simulink model "controller"  (R2018a)
settings: Solver=FixedStepAuto  StartTime=0.0  StopTime=inf  FixedStep=0.02  RelTol=1e-3  EnableMultiTasking=on
values from neighbouring files (symbols this model uses):
  data = zeros(2,4)    [LaneCal.m]
undefined symbols (not defined in the file or in its folder): control
libraries: simulink x21
settings Model: SimulationMode=accelerator  Creator=Owen  LastModifiedBy=shun.yang
settings SolverCC: AutoInsertRateTranBlk=on
settings DataIOCC: LimitDataPoints=on  SaveFormat=Array
settings OptimizationCC: EfficientMapNaN2IntZero=off  LifeSpan=inf  AccelVerboseBuild=on
settings DebuggingCC: SolverPrmCheckMsg=warning  SFUnexpectedBacktrackingDiag=warning  SFNoUnconditionalDefaultTransitionDiag=warning  SFExecutionAtInitializationDiag=none
settings HardwareCC: ProdBitPerPointer=32  ProdBitPerSizeT=32  ProdBitPerPtrDiffT=32  ProdLargestAtomicFloat=None  ProdIntDivRoundTo=Undefined  ProdEndianess=Unspecified  ProdWordSize=32  ProdHWDeviceType=32-bit Generic  TargetBitPerPointer=64  TargetBitPerSizeT=64  TargetBitPerPtrDiffT=64  TargetLongLongMode=on  TargetIntDivRoundTo=Zero  TargetEndianess=LittleEndian  TargetWordSize=64  TargetHWDeviceType=MATLAB Host  ProdEqTarget=off
settings ModelReferenceCC: PropagateSignalLabelsOutOfModel=off
settings SFSimCC: SimCustomInitializer=initTORCSLink();  SimCustomTerminator=terminateTORCSLink();  SimUserSources=TORCSLink.c  SimBuildMode=sf_nonincremental_build  SimGenImportedTypeDefs=on
settings CodeAppCC: MaxIdLength=128  StateflowObjectComments=on
settings GRTTargetCC: TargetLangStandard=C89/C90 (ANSI)  GeneratePreprocessorConditionals=Disable all  CombineOutputUpdateFcns=off  GRTInterface=on
settings ConfigComp: CovMetricSettings=dw  CovHtmlReporting=on  CovSaveCumulativeToWorkspaceVar=on  CovSaveSingleToWorkspaceVar=on  CovExternalEMLEnable=off  CovSFcnEnable=off

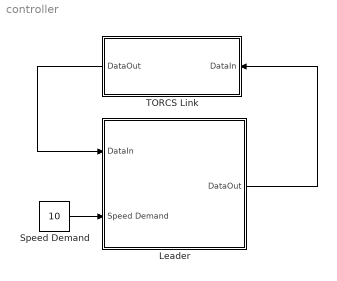
== system controller ==
  Leader : Subsystem
  Speed Demand : Constant  Value=10
  TORCS Link : Subsystem  LoadFcn=|  InitFcn=|
      LoadFcn=|
      | load VehicleBusses.mat;
      | src = 'TORCSLink.c';
      | init = 'initTORCSLink();';
      | term = 'terminateTORCSLink();';
      | simSrc = get_param(gcs,'SimUserSources');
      | simInit = get_param(gcs,'SimCustomInitializer');
      | simTerm = get_param(gcs,'SimCustomTerminator');
      | 
      | if isempty(strfind(simSrc,src))
      |   fprintf('Adding %s to Custom Sources\n', src);
      |   set_param(gcs,'SimUserSources', [simSrc 10 src]);
      | end
      | 
      | if isempty(strfind(simInit,init))
      |   fprintf('Adding %s to Custom Initialisation Code\n', init);
      |   set_param(gcs,'SimCustomInitializer', [simInit 10 init]);
      | end
      | 
      | if isempty(strfind(simTerm,term))
      |   fprintf('Adding %s to Custom Termination Code\n', term);
      |   set_param(gcs,'SimCustomTerminator', [simTerm 10 term]);
      | end
      | 
      | if isunix
      |     libs = 'librt.so';
      |     simLibs = get_param(gcs,'SimUserLibraries');
      | 
      |     if isempty(strfind(simLibs,libs))
      |       fprintf('Adding %s to Custom Libraries\n', libs);
      |       set_param(gcs,'SimUserLibraries', [simLibs 10 libs]);
      |     end
      | else
      |    set_param(gcs,'SimUserLibraries', '');
      | end
      | 
      | clear src init term simSrc simInit simTerm libs simLibs;
      InitFcn=|
      | load VehicleBusses.mat;
      | src = 'TORCSLink.c';
      | init = 'initTORCSLink();';
      | term = 'terminateTORCSLink();';
      | simSrc = get_param(gcs,'SimUserSources');
      | simInit = get_param(gcs,'SimCustomInitializer');
      | simTerm = get_param(gcs,'SimCustomTerminator');
      | 
      | if isempty(strfind(simSrc,src))
      |   fprintf('Adding %s to Custom Sources\n', src);
      |   set_param(gcs,'SimUserSources', [simSrc 10 src]);
      | end
      | 
      | if isempty(strfind(simInit,init))
      |   fprintf('Adding %s to Custom Initialisation Code\n', init);
      |   set_param(gcs,'SimCustomInitializer', [simInit 10 init]);
      | end
      | 
      | if isempty(strfind(simTerm,term))
      |   fprintf('Adding %s to Custom Termination Code\n', term);
      |   set_param(gcs,'SimCustomTerminator', [simTerm 10 term]);
      | end
      | 
      | if isunix
      |     libs = 'librt.so';
      |     simLibs = get_param(gcs,'SimUserLibraries');
      | 
      |     if isempty(strfind(simLibs,libs))
      |       fprintf('Adding %s to Custom Libraries\n', libs);
      |       set_param(gcs,'SimUserLibraries', [simLibs 10 libs]);
      |     end
      | else
      |    set_param(gcs,'SimUserLibraries', '');
      | end
      | 
      | clear src init term simSrc simInit simTerm libs simLibs;
  wires:
  TORCS Link/1(DataOut) -> Leader/1(DataIn)
  Speed Demand/1 -> Leader/2(Speed Demand)
  Leader/1(DataOut) -> TORCS Link/1(DataIn)

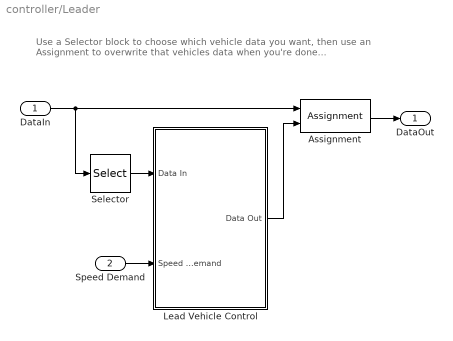
== system controller/Leader ==
  note: Use a Selector block to choose which vehicle data you want,
      | then use an Assignment to overwrite that vehicles data when you're done...
  DataIn : Inport
  Speed Demand : Inport  Port=2
  Assignment : Assignment  DiagnosticForDimensions=Warning  IndexOptions=Index vector (dialog)  Indices=1  OutputSizes=1
  Lead Vehicle Control : Subsystem  InitFcn=run Inita.m
  Selector : Selector  InputPortWidth=10  IndexOptions=Index vector (dialog)  Indices=1  OutputSizes=1
  DataOut : Outport
  wires:
  Speed Demand/1 -> Lead Vehicle Control/2(Speed Demand)
  DataIn/1 -> Selector/1, Assignment/1
  Selector/1 -> Lead Vehicle Control/1(Data In)
  Assignment/1 -> DataOut/1
  Lead Vehicle Control/1(Data Out) -> Assignment/2

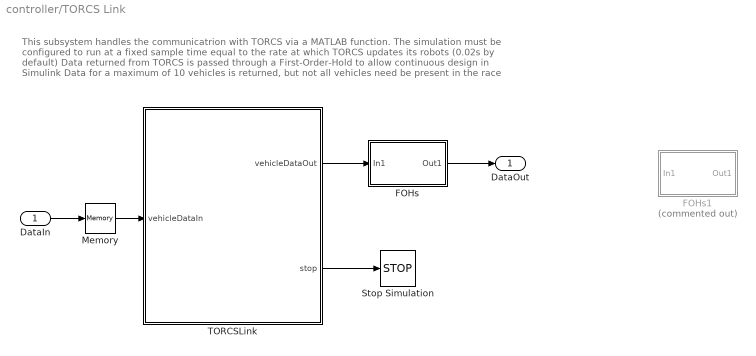
== system controller/TORCS Link ==
  note: This subsystem handles the communicatrion with TORCS via a MATLAB function.
      | The simulation must be configured to run at a fixed sample time equal to the rate at which TORCS updates its robots (0.02s by default)
      | Data returned from TORCS is passed through a First-Order-Hold to allow continuous design in Simulink
      | Data for a maximum of 10 vehicles is returned, but not all vehicles need be present in the race
  DataIn : Inport
  FOHs : Subsystem  TreatAsAtomicUnit=on
  FOHs1 : Subsystem  Commented=on  TreatAsAtomicUnit=on
  Memory : Memory
  Stop Simulation : Stop
  TORCSLink : MATLAB Function  TreatAsAtomicUnit=on
  DataOut : Outport
  wires:
  Memory/1 -> TORCSLink/1(vehicleDataIn)
  DataIn/1 -> Memory/1
  TORCSLink/2(stop) -> Stop Simulation/1
  TORCSLink/1(vehicleDataOut) -> FOHs/1(In1)
  FOHs/1(Out1) -> DataOut/1

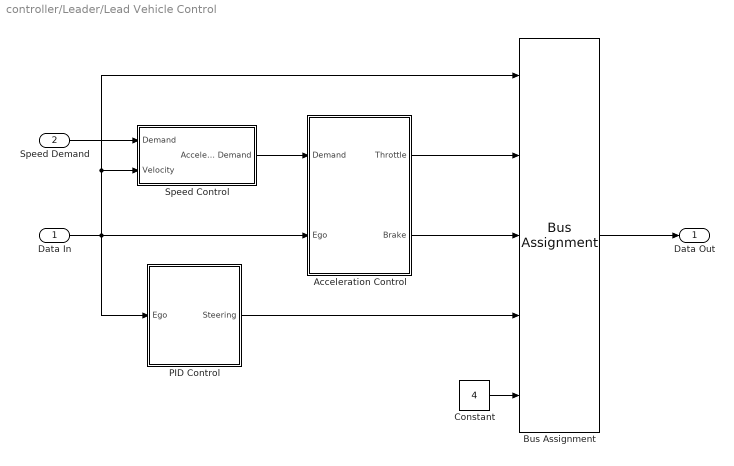
== system controller/Leader/Lead Vehicle Control ==
  Data In : Inport
  Speed Demand : Inport  Port=2
  Acceleration Control : Subsystem
  Bus Assignment : BusAssignment  AssignedSignals=control.throttle,control.brake,control.steering,control.gear
  Constant : Constant  Value=4  OutDataTypeStr=int32
  PID Control : Subsystem
  Speed Control : Subsystem
  Data Out : Outport
  wires:
  Speed Demand/1 -> Speed Control/1(Demand)
  Bus Assignment/1 -> Data Out/1
  Speed Control/1(Acceleration Demand) -> Acceleration Control/1(Demand)
  Data In/1 -> Acceleration Control/2(Ego), PID Control/1(Ego), Speed Control/2(Velocity), Bus Assignment/1
  Acceleration Control/2(Brake) -> Bus Assignment/3
  Acceleration Control/1(Throttle) -> Bus Assignment/2
  Constant/1 -> Bus Assignment/5
  PID Control/1(Steering) -> Bus Assignment/4

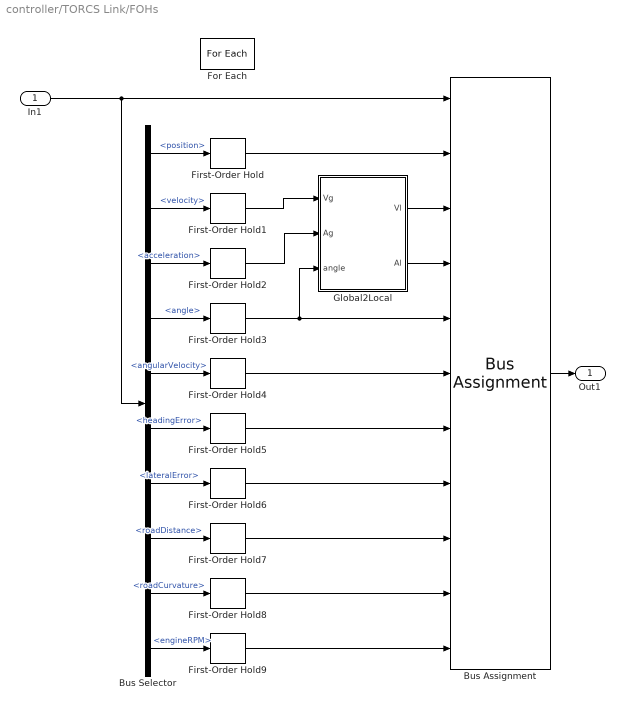
== system controller/TORCS Link/FOHs ==
  In1 : Inport  Partition=on  PartitionDimension=1  PartitionWidth=1  PartitionOffset=0
  Bus Assignment : BusAssignment  AssignedSignals=data.position,data.velocity,data.acceleration,data.angle,data.angularVelocity,data.headingError,data.lateralError,data.roadDistance,data.roadCurvature,data.engineRPM
  Bus Selector : BusSelector  OutputSignals=data.position,data.velocity,data.acceleration,data.angle,data.angularVelocity,data.headingError,data.lateralError,data.roadDistance,data.roadCurvature,data.engineRPM
  First-Order Hold{,1..9} (10 alike) : simulink/Discrete/First-Order Hold  DisableCoverage=on  Ts=0.02
      settings: SourceProductName=Simulink  SourceProductBaseCode=SL
  For Each : ForEach  DisableCoverage=on  IndexMode=One-based
  Global2Local : MATLAB Function  TreatAsAtomicUnit=on
  Out1 : Outport  ConcatenationDimension=1
  wires:
  Bus Assignment/1 -> Out1/1
  Bus Selector/10 -> First-Order Hold9/1  "<engineRPM>"
  Bus Selector/9 -> First-Order Hold8/1  "<roadCurvature>"
  Bus Selector/8 -> First-Order Hold7/1  "<roadDistance>"
  Bus Selector/7 -> First-Order Hold6/1  "<lateralError>"
  Bus Selector/6 -> First-Order Hold5/1  "<headingError>"
  Bus Selector/5 -> First-Order Hold4/1  "<angularVelocity>"
  Bus Selector/3 -> First-Order Hold2/1  "<acceleration>"
  Bus Selector/2 -> First-Order Hold1/1  "<velocity>"
  Bus Selector/1 -> First-Order Hold/1  "<position>"
  In1/1 -> Bus Assignment/1, Bus Selector/1
  Bus Selector/4 -> First-Order Hold3/1  "<angle>"
  First-Order Hold3/1 -> Global2Local/3(angle), Bus Assignment/5
  First-Order Hold4/1 -> Bus Assignment/6
  First-Order Hold5/1 -> Bus Assignment/7
  First-Order Hold6/1 -> Bus Assignment/8
  First-Order Hold7/1 -> Bus Assignment/9
  First-Order Hold8/1 -> Bus Assignment/10
  First-Order Hold9/1 -> Bus Assignment/11
  First-Order Hold1/1 -> Global2Local/1(Vg)
  First-Order Hold2/1 -> Global2Local/2(Ag)
  First-Order Hold/1 -> Bus Assignment/2
  Global2Local/2(Al) -> Bus Assignment/4
  Global2Local/1(Vl) -> Bus Assignment/3

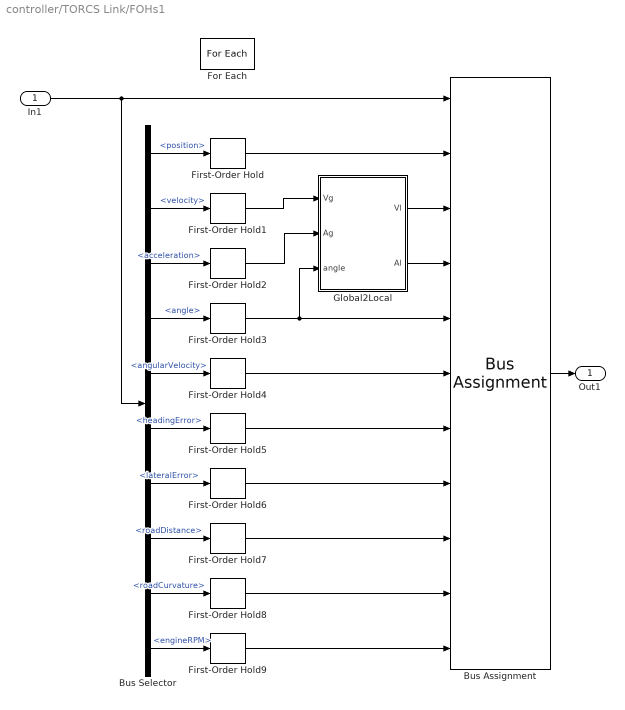
== system controller/TORCS Link/FOHs1 ==
  In1 : Inport  Partition=on  PartitionDimension=1  PartitionWidth=1  PartitionOffset=0
  Bus Assignment : BusAssignment  AssignedSignals=data.position,data.velocity,data.acceleration,data.angle,data.angularVelocity,data.headingError,data.lateralError,data.roadDistance,data.roadCurvature,data.engineRPM
  Bus Selector : BusSelector  OutputSignals=data.position,data.velocity,data.acceleration,data.angle,data.angularVelocity,data.headingError,data.lateralError,data.roadDistance,data.roadCurvature,data.engineRPM
  First-Order Hold{,1..9} (10 alike) : simulink/Discrete/First-Order Hold  DisableCoverage=on  Ts=0.1
      settings: SourceProductName=Simulink  SourceProductBaseCode=SL
  For Each : ForEach  DisableCoverage=on  IndexMode=One-based
  Global2Local : MATLAB Function  TreatAsAtomicUnit=on
  Out1 : Outport  ConcatenationDimension=1
  wires:
  Global2Local/1(Vl) -> Bus Assignment/3
  Global2Local/2(Al) -> Bus Assignment/4
  First-Order Hold/1 -> Bus Assignment/2
  First-Order Hold2/1 -> Global2Local/2(Ag)
  First-Order Hold1/1 -> Global2Local/1(Vg)
  First-Order Hold9/1 -> Bus Assignment/11
  First-Order Hold8/1 -> Bus Assignment/10
  First-Order Hold7/1 -> Bus Assignment/9
  First-Order Hold6/1 -> Bus Assignment/8
  First-Order Hold5/1 -> Bus Assignment/7
  First-Order Hold4/1 -> Bus Assignment/6
  First-Order Hold3/1 -> Bus Assignment/5, Global2Local/3(angle)
  Bus Selector/4 -> First-Order Hold3/1  "<angle>"
  In1/1 -> Bus Selector/1, Bus Assignment/1
  Bus Selector/1 -> First-Order Hold/1  "<position>"
  Bus Selector/2 -> First-Order Hold1/1  "<velocity>"
  Bus Selector/3 -> First-Order Hold2/1  "<acceleration>"
  Bus Selector/5 -> First-Order Hold4/1  "<angularVelocity>"
  Bus Selector/6 -> First-Order Hold5/1  "<headingError>"
  Bus Selector/7 -> First-Order Hold6/1  "<lateralError>"
  Bus Selector/8 -> First-Order Hold7/1  "<roadDistance>"
  Bus Selector/9 -> First-Order Hold8/1  "<roadCurvature>"
  Bus Selector/10 -> First-Order Hold9/1  "<engineRPM>"
  Bus Assignment/1 -> Out1/1

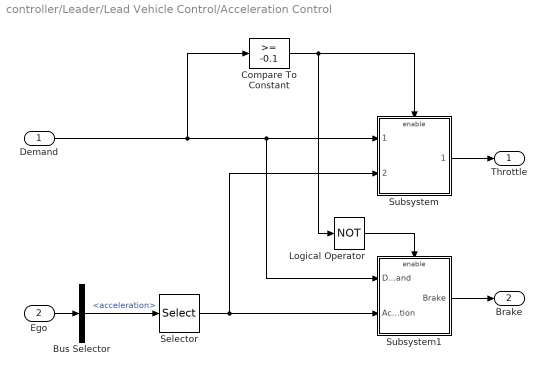
== system controller/Leader/Lead Vehicle Control/Acceleration Control ==
  Demand : Inport
  Ego : Inport  Port=2
  Bus Selector : BusSelector  OutputSignals=data.acceleration
  Compare To Constant : simulink/Logic and Bit Operations/Compare To Constant  relop=>=  const=-0.1  OutDataTypeStr=boolean
  Logical Operator : Logic  Operator=NOT  AllPortsSameDT=off  OutDataTypeStr=boolean
  Selector : Selector  InputPortWidth=3  IndexOptions=Index vector (dialog)  Indices=1  OutputSizes=1
  Subsystem : Subsystem
  Subsystem1 : Subsystem
  Throttle : Outport
  Brake : Outport  Port=2
  wires:
  Selector/1 -> Subsystem/2(Acceleration), Subsystem1/2(Acceleration)
  Demand/1 -> Compare To Constant/1, Subsystem1/1(Demand), Subsystem/1(Demand)
  Subsystem1/1(Brake) -> Brake/1
  Subsystem/1(Throttle) -> Throttle/1
  Compare To Constant/1 -> Subsystem/Enable, Logical Operator/1
  Logical Operator/1 -> Subsystem1/Enable
  Ego/1 -> Bus Selector/1
  Bus Selector/1 -> Selector/1  "<acceleration>"

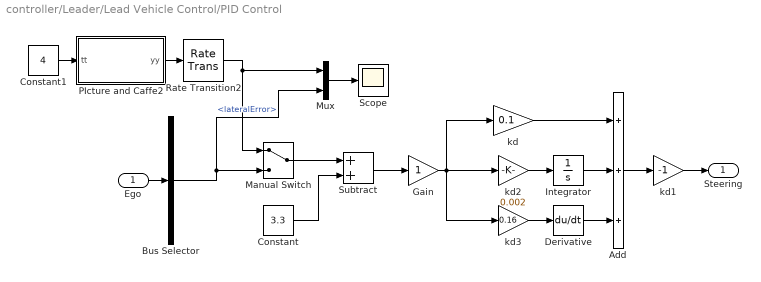
== system controller/Leader/Lead Vehicle Control/PID Control ==
  Ego : Inport
  Add : Sum  Inputs=3
  Bus Selector : BusSelector  OutputSignals=data.lateralError
  Constant : Constant  Value=3.3
  Constant1 : Constant  Value=4  OutDataTypeStr=int32  SampleTime=0.2
  Derivative : Derivative
  Gain : Gain
  Integrator : Integrator
  Manual Switch : ManualSwitch
  Mux : Mux  Inputs=2
  PIcture and Caffe2 : MATLAB Function  TreatAsAtomicUnit=on
  Rate Transition2 : RateTransition  Deterministic=off  OutPortSampleTime=0.02
  Scope : Scope
  Subtract : Sum
  kd : Gain  Gain=0.1
  kd1 : Gain  Gain=-1
  kd2 : Gain  Gain=0.002
  kd3 : Gain  Gain=0.16
  Steering : Outport
  wires:
  Ego/1 -> Bus Selector/1
  Constant/1 -> Subtract/2
  Subtract/1 -> Gain/1
  kd1/1 -> Steering/1
  kd/1 -> Add/1
  kd2/1 -> Integrator/1
  Integrator/1 -> Add/2
  Derivative/1 -> Add/3
  kd3/1 -> Derivative/1
  Gain/1 -> kd3/1, kd/1, kd2/1
  Add/1 -> kd1/1
  Bus Selector/1 -> Mux/2, Manual Switch/2  "<lateralError>"
  Manual Switch/1 -> Subtract/1
  Constant1/1 -> PIcture and Caffe2/1(tt)
  Mux/1 -> Scope/1
  PIcture and Caffe2/1(yy) -> Rate Transition2/1
  Rate Transition2/1 -> Manual Switch/1, Mux/1

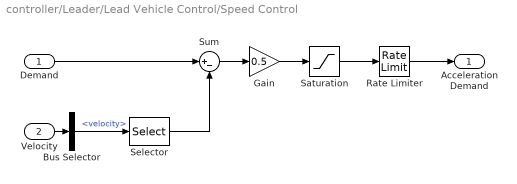
== system controller/Leader/Lead Vehicle Control/Speed Control ==
  Demand : Inport
  Velocity : Inport  Port=2
  Bus Selector : BusSelector  OutputSignals=data.velocity
  Gain : Gain  Gain=0.5
  Rate Limiter : RateLimiter  RisingSlewLimit=inf  FallingSlewLimit=-inf  SampleTimeMode=inherited
  Saturation : Saturate  UpperLimit=2  LowerLimit=-4
  Selector : Selector  InputPortWidth=3  IndexOptions=Index vector (dialog)  Indices=1  OutputSizes=1
  Sum : Sum  Inputs=|+-
  Acceleration Demand : Outport
  wires:
  Gain/1 -> Saturation/1
  Sum/1 -> Gain/1
  Demand/1 -> Sum/1
  Saturation/1 -> Rate Limiter/1
  Selector/1 -> Sum/2
  Rate Limiter/1 -> Acceleration Demand/1
  Velocity/1 -> Bus Selector/1
  Bus Selector/1 -> Selector/1  "<velocity>"

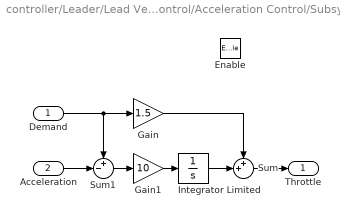
== system controller/Leader/Lead Vehicle Control/Acceleration Control/Subsystem ==
  Demand : Inport
  Acceleration : Inport  Port=2
  Enable : EnablePort  StatesWhenEnabling=reset
  Gain : Gain  Gain=1.5
  Gain1 : Gain  Gain=10
  Integrator Limited : Integrator  LimitOutput=on  UpperSaturationLimit=1  LowerSaturationLimit=-1
  Sum : Sum  Inputs=++|
  Sum1 : Sum  Inputs=+-|
  Throttle : Outport  OutputWhenDisabled=reset  InitialOutput=0
  wires:
  Gain/1 -> Sum/1
  Integrator Limited/1 -> Sum/2
  Gain1/1 -> Integrator Limited/1
  Sum/1 -> Throttle/1
  Demand/1 -> Sum1/1, Gain/1
  Acceleration/1 -> Sum1/2
  Sum1/1 -> Gain1/1

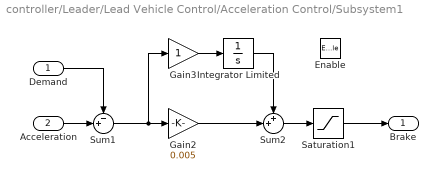
== system controller/Leader/Lead Vehicle Control/Acceleration Control/Subsystem1 ==
  Demand : Inport
  Acceleration : Inport  Port=2
  Enable : EnablePort  StatesWhenEnabling=reset
  Gain2 : Gain  Gain=0.005
  Gain3 : Gain
  Integrator Limited : Integrator  LimitOutput=on  UpperSaturationLimit=1  LowerSaturationLimit=-1
  Saturation1 : Saturate  UpperLimit=1  LowerLimit=0
  Sum1 : Sum  Inputs=-+|
  Sum2 : Sum  Inputs=++|
  Brake : Outport  OutputWhenDisabled=reset  InitialOutput=0
  wires:
  Saturation1/1 -> Brake/1
  Sum2/1 -> Saturation1/1
  Gain2/1 -> Sum2/2
  Integrator Limited/1 -> Sum2/1
  Gain3/1 -> Integrator Limited/1
  Sum1/1 -> Gain2/1, Gain3/1
  Demand/1 -> Sum1/1
  Acceleration/1 -> Sum1/2

== matlab function controller/TORCS Link/TORCSLink ==
  data: vehicleDataIn input Bus: VehicleBus size=10; vehicleDataOut output Bus: VehicleBus size=10; stop output
function [vehicleDataOut, stop] = TORCSLink(vehicleDataIn)
%#codegen
stop = 0;
flag = int32(0);

% Simulink doesn't like passing the array of structures to C function (no
% idea why?!), so we have to seperate out the three stages

% Update vehicle control values in TORCS
for i=1:10
    flag = coder.ceval('setVehicleControl', int32(i-1), vehicleDataIn(i).control);
    if (flag < 0)
        fprintf('No connection to TORCS!\n');
        stop = 1;
    end
end

% Tell TORCS it can update (this function hangs until new data is
% available)
flag = coder.ceval('updateTORCS');
if (flag < 0)
    fprintf('No data from TORCS! (%d) \n', flag);
    stop = 1;
end

% Read in new data from TORCS
for i=1:10
    % Can't pass this directly to coder.ref
    data = vehicleDataIn(i).data;
    flag = coder.ceval('getVehicleData', int32(i-1), coder.ref(data));
    vehicleDataIn(i).data = data;
    if (flag < 0)
        fprintf('No connection to TORCS!\n');
        stop = 1;
    end
end

vehicleDataOut = vehicleDataIn;

== matlab function controller/TORCS Link/FOHs/Global2Local ==
  data: Vg input; Ag input; angle input; Vl output; Al output
function [Vl,Al] = fcn(Vg,Ag,angle)
%#codegen

phi=angle(3);
R = [cos(phi) sin(phi) 0; -sin(phi) cos(phi) 0; 0 0 1];

Vl = R*Vg;
Al = R*Ag;

== matlab function controller/TORCS Link/FOHs1/Global2Local ==
  data: Vg input; Ag input; angle input; Vl output; Al output
function [Vl,Al] = fcn(Vg,Ag,angle)
%#codegen

phi=angle(3);
R = [cos(phi) sin(phi) 0; -sin(phi) cos(phi) 0; 0 0 1];

Vl = R*Vg;
Al = R*Ag;

== matlab function controller/Leader/Lead Vehicle Control/PID Control/PIcture and Caffe2 ==
  data: yy output; tt input
function yy=captureScreen(tt)

    coder.extrinsic('LaneCal')
    yy=zeros(1);
    yy = LaneCal();

end
